simulink model "virtual_world_first_scenario_modified_1"  (R2015b)
settings: Solver=VariableStepAuto  StartTime=start_time  StopTime=stop_time  RelTol=1e-3
values from neighbouring files (symbols this model uses):
  colorFirstCar = [255 0 0]    [virtual_world_script.m]
  colorSecondCar = [0.88 0.95 0.0]    [virtual_world_script.m]
  distanceAmongCars = [0 0 2]    [virtual_world_script.m]
  observer_position = [z_pross y_pross x_pross]    [simulazione_sistema.m]    (also in virtual_world.m = [z_next y_next x_next]; virtual_world_script.m = [z_next y_next x_next])
  rotation_matrix = R_1 * R_2 * R_3    [simulazione_sistema.m]    (also in virtual_world.m = R_z * R_y * R_x; virtual_world_script.m = R_z * R_y * R_x)
  simulationStep = 0.05    [simulation_parameters.m]
libraries: vrlib x50, visionsinks x1
settings Model: ExtModeArmWhenConnect=off  Creator=Giuseppe Silano  LastModifiedBy=giuse
settings DataIOCC: SaveFormat=Array  SignalLoggingName=sigsOut
settings OptimizationCC: BooleanDataType=off  OptimizeBlockIOStorage=off  BufferReuse=off  GlobalBufferReuse=off  ExpressionFolding=off  ExpressionDepthLimit=2147483647  LocalBlockOutputs=off  InitFltsAndDblsToZero=on
settings DebuggingCC: UnderspecifiedInitializationDetection=Classic  MergeDetectMultiDrivingBlocksExec=none  CheckExecutionContextPreStartOutputMsg=on  CheckExecutionContextRuntimeOutputMsg=on  SignalResolutionControl=TryResolveAllWithWarning  MultiTaskDSMMsg=warning  MultiTaskCondExecSysMsg=none  FcnCallInpInsideContextMsg=UseLocalSettings  StateNameClashWarn=warning
settings HardwareCC: ProdBitPerPointer=32  ProdLargestAtomicFloat=None  ProdIntDivRoundTo=Undefined  ProdEndianess=Unspecified  ProdWordSize=32  ProdHWDeviceType=32-bit Generic
settings RTWCC: RetainRTWFile=on
settings GRTTargetCC: TargetFcnLib=ansi_tfl_tmw.mat  GeneratePreprocessorConditionals=Disable all  CombineOutputUpdateFcns=off  GRTInterface=on
settings ConfigComp: CovModelRefEnable=Off  CovSFcnEnable=off

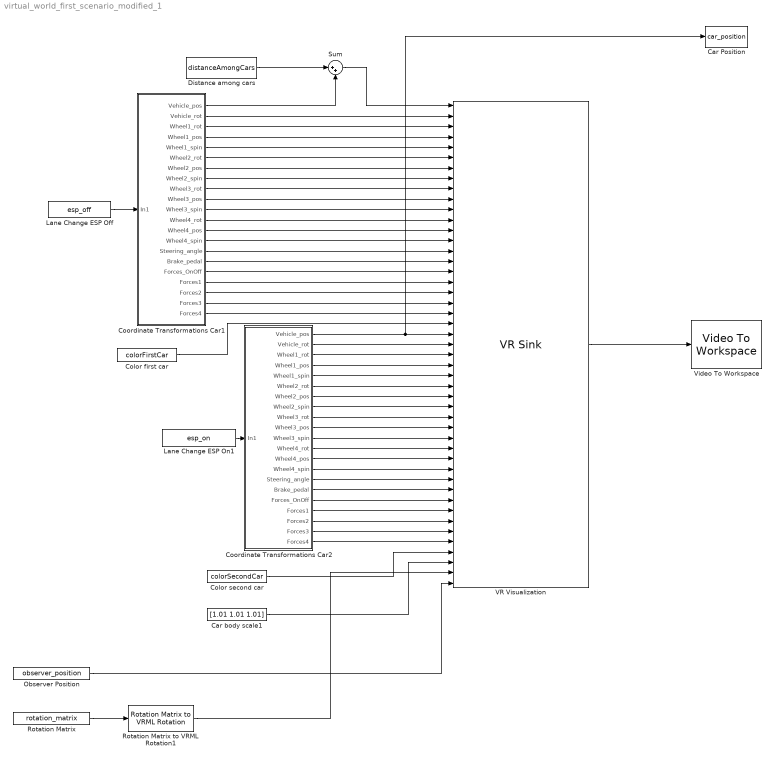
== system virtual_world_first_scenario_modified_1 ==
  Car Position : ToWorkspace  VariableName=car_position  SampleTime=-1
      settings: MaxDataPoints=1
  Car body scale1 : Constant  Value=[1.01 1.01 1.01]
  Color first car : Constant  Value=colorFirstCar
  Color second car : Constant  Value=colorSecondCar
  Coordinate Transformations Car1 : Subsystem
  Coordinate Transformations Car2 : Subsystem
  Distance among cars : Constant  Value=distanceAmongCars
  Lane Change ESP On1 : FromWorkspace  VariableName=esp_on  SampleTime=simulationStep  OutputAfterFinalValue=Holding final value
  "Lane Change ESP Off " : FromWorkspace  VariableName=esp_off  SampleTime=simulationStep  OutputAfterFinalValue=Holding final value
  Observer Position : Constant  Value=observer_position
  Rotation Matrix : Constant  Value=rotation_matrix
  Rotation Matrix to VRML Rotation1 : vrlib/Utilities/Rotation Matrix to VRML Rotation  maxzero=1e-12
  Sum : Sum  Inputs=|++
  VR Visualization : vrlib/VR Sink  InstantiateOnLoad=on  SampleTime=-1  ViewEnable=on  RemoteChange=off  RemoteView=on  FieldsWritten=Car_1.Car_Position.3.1.1.double#Car_1.Car_Rotation.4.1.1.double#Car_1.WheelFL_Rotation.4.1.1.double#Car_1.WheelFL_Translation.3.1.1.double#Car_1.WheelFL_Spin_Rotation.4.1.1.double#Car_1.WheelFR_Rotation.4.1.1.double#Car_1.WheelFR_Translation.3.1.1.double#Car_1.WheelFR_Spin_Rotation.4.1.1.double#Car_1.WheelRL_Rotation.4.1.1.double#Car_1.WheelRL_Translation.3.1.1.double#Car_1.WheelRL_Spin_Rotation.4.1.1.double#Car_1.WheelRR_Rotation.4.1.1.double#Car_1.WheelRR_Translation.3.1.1.double#Car_1.WheelRR_Spin_Rotation.4.1.1.double#Car_1.SteeringWheel1_Rotation.4.1.1.double#Car_1.Backlights_Switch.1.1.1.double#Car_1.Forces_Switch.1.1.1.double#Car_1.Force1_Scale.3.1.1.double#Car_1.Force2_Scale.3.1.1.double#Car_1.Force3_Scale.3.1.1.double#Car_1.Force4_Scale.3.1.1.double#Car_1.Car_DiffuseColor.3.1.1.double#Car_2.Car_Position.3.1.1.double#Car_2.Car_Rotation.4.1.1.double#Car_2.WheelFL_Rotation.4.1.1.double#Car_2.WheelFL_Translation.3.1.1.double#Car_2.WheelFL_Spin_Rotation.4.1.1.double#Car_2.WheelFR_Rotation.4.1.1.double#Car_2.WheelFR_Translation.3.1.1.double#Car_2.WheelFR_Spin_Rotation.4.1.1.double#Car_2.WheelRL_Rotation.4.1.1.double#Car_2.WheelRL_Translation.3.1.1.double#Car_2.WheelRL_Spin_Rotation.4.1.1.double#Car_2.WheelRR_Rotation.4.1.1.double#Car_2.WheelRR_Translation.3.1.1.double#Car_2.WheelRR_Spin_Rotation.4.1.1.double#Car_2.SteeringWheel1_Rotation.4.1.1.double#Car_2.Backlights_Switch.1.1.1.double#Car_2.Forces_Switch.1.1.1.double#Car_2.Force1_Scale.3.1.1.double#Car_2.Force2_Scale.3.1.1.double#Car_2.Force3_Scale.3.1.1.double#Car_2.Force4_Scale.3.1.1.double#Car_2.Car_DiffuseColor.3.1.1.double#Car_2.Body_Scale.3.1.1.double#FlyingCamera.orientation.4.1.1.double#FlyingCamera.position.3.1.1.double  WorldFileName=octavia_scene_lchg_2cars_modified_scenario_1.wrl  WorldDescription=Vehicle Dynamics Visualization - Multiple Vehicles  AutoView=on  VideoDimensions=[800 600]  AllowVariableSize=off  FigureProperties="{'Position', 'Name', 'Viewpoint', 'CameraBound', 'CameraDirection', 'CameraPosition', 'CameraUpVector', 'ZoomFactor', 'Antialiasing', 'Headlight', 'Lighting', 'NavPanel', 'Sound', 'StatusBar', 'Stereo3D', 'Stereo3DCameraOffset', 'Stereo3DHIT', 'ToolBar', 'Textures', 'Transparency', 'Triad', 'Wireframe', 'NavZones', 'NavMode', 'NavSpeed', 'CaptureFileFormat', 'CaptureFileName', 'Record2DCompressMethod', 'Record2DCompressQuality', 'Record2D', 'Record2DFileName', 'Record2DFPS'; [1.5200000000000000e+02   2.4800000000000000e+02   5.7600000000000000e+02   3.8000000000000000e+02], 'Vehicle Dynamics Visualization - Multiple Vehicles', 'Car - View from Right Above Ahead', 'on', [0.0000000000000000e+00   0.0000000000000000e+00  -1.0000000000000000e+00], [0.0000000000000000e+00   0.0000000000000000e+00   0.0000000000000000e+00], [0.0000000000000000e+00   1.0000000000000000e+00   0.0000000000000000e+00], [1.0000000000000000e+00], 'on', 'off', 'on', 'halfbar', 'on', 'on', 'off', [1.0000000149011612e-01], [0.0000000000000000e+00], 'on', 'on', 'on', 'none', 'off', 'off', 'walk', 'normal', 'tif', '%f_anim_%n.tif', 'auto', [7.5000000000000000e+01], 'off', '%f_anim_%n.avi', 'auto'; [7.3300000000000000e+02   6.0000000000000000e+01   6.0000000000000000e+02   8.0000000000000000e+02], 'Vehicle Dynamics Visualization - Multiple Vehicles', 'External observer: drone', 'on', [0.0000000000000000e+00   0.0000000000000000e+00  -1.0000000000000000e+00], [0.0000000000000000e+00   0.0000000000000000e+00   0.0000000000000000e+00], [0.0000000000000000e+00   1.0000000000000000e+00   0.0000000000000000e+00], [1.0000000000000000e+00], 'on', 'off', 'on', 'none', 'on', 'off', 'off', [1.0000000149011612e-01], [0.0000000000000000e+00], 'off', 'on', 'on', 'none', 'off', 'off', 'walk', 'normal', 'tif', '%f_anim_%n.tif', 'auto', [7.5000000000000000e+01], 'off', '***video***', 'auto'}"
  Video To Workspace : visionsinks/Video To Workspace  VariableName=image  NumInputs=1  DataLimit=1  DecimationFactor=1  LogFi=off  InPortLabels=R|G|B
  wires:
  VR Visualization/1 -> Video To Workspace/1
  "Lane Change ESP Off "/1 -> Coordinate Transformations Car1/1(In1)
  Lane Change ESP On1/1 -> Coordinate Transformations Car2/1(In1)
  Rotation Matrix/1 -> Rotation Matrix to VRML Rotation1/1
  Distance among cars/1 -> Sum/1
  Coordinate Transformations Car1/2(Vehicle_rot) -> VR Visualization/2
  Coordinate Transformations Car1/3(Wheel1_rot) -> VR Visualization/3
  Coordinate Transformations Car1/4(Wheel1_pos) -> VR Visualization/4
  Coordinate Transformations Car1/5(Wheel1_spin) -> VR Visualization/5
  Coordinate Transformations Car1/6(Wheel2_rot) -> VR Visualization/6
  Coordinate Transformations Car1/7(Wheel2_pos) -> VR Visualization/7
  Coordinate Transformations Car1/8(Wheel2_spin) -> VR Visualization/8
  Coordinate Transformations Car1/9(Wheel3_rot) -> VR Visualization/9
  Coordinate Transformations Car1/10(Wheel3_pos) -> VR Visualization/10
  Coordinate Transformations Car1/11(Wheel3_spin) -> VR Visualization/11
  Coordinate Transformations Car1/12(Wheel4_rot) -> VR Visualization/12
  Coordinate Transformations Car1/13(Wheel4_pos) -> VR Visualization/13
  Coordinate Transformations Car1/14(Wheel4_spin) -> VR Visualization/14
  Coordinate Transformations Car1/15(Steering_angle) -> VR Visualization/15
  Coordinate Transformations Car1/16(Brake_pedal) -> VR Visualization/16
  Coordinate Transformations Car1/17(Forces_OnOff) -> VR Visualization/17
  Coordinate Transformations Car1/18(Forces1) -> VR Visualization/18
  Coordinate Transformations Car1/19(Forces2) -> VR Visualization/19
  Coordinate Transformations Car1/20(Forces3) -> VR Visualization/20
  Coordinate Transformations Car1/21(Forces4) -> VR Visualization/21
  Color first car/1 -> VR Visualization/22
  Coordinate Transformations Car2/2(Vehicle_rot) -> VR Visualization/24
  Coordinate Transformations Car2/3(Wheel1_rot) -> VR Visualization/25
  Coordinate Transformations Car2/4(Wheel1_pos) -> VR Visualization/26
  Coordinate Transformations Car2/5(Wheel1_spin) -> VR Visualization/27
  Coordinate Transformations Car2/6(Wheel2_rot) -> VR Visualization/28
  Coordinate Transformations Car2/7(Wheel2_pos) -> VR Visualization/29
  Coordinate Transformations Car2/8(Wheel2_spin) -> VR Visualization/30
  Coordinate Transformations Car2/9(Wheel3_rot) -> VR Visualization/31
  Coordinate Transformations Car2/10(Wheel3_pos) -> VR Visualization/32
  Coordinate Transformations Car2/11(Wheel3_spin) -> VR Visualization/33
  Coordinate Transformations Car2/12(Wheel4_rot) -> VR Visualization/34
  Coordinate Transformations Car2/13(Wheel4_pos) -> VR Visualization/35
  Coordinate Transformations Car2/14(Wheel4_spin) -> VR Visualization/36
  Coordinate Transformations Car2/15(Steering_angle) -> VR Visualization/37
  Coordinate Transformations Car2/16(Brake_pedal) -> VR Visualization/38
  Coordinate Transformations Car2/17(Forces_OnOff) -> VR Visualization/39
  Coordinate Transformations Car2/18(Forces1) -> VR Visualization/40
  Coordinate Transformations Car2/19(Forces2) -> VR Visualization/41
  Coordinate Transformations Car2/20(Forces3) -> VR Visualization/42
  Coordinate Transformations Car2/21(Forces4) -> VR Visualization/43
  Color second car/1 -> VR Visualization/44
  Car body scale1/1 -> VR Visualization/45
  Rotation Matrix to VRML Rotation1/1 -> VR Visualization/46
  Observer Position/1 -> VR Visualization/47
  Coordinate Transformations Car2/1(Vehicle_pos) -> Car Position/1, VR Visualization/23
  Coordinate Transformations Car1/1(Vehicle_pos) -> Sum/2
  Sum/1 -> VR Visualization/1

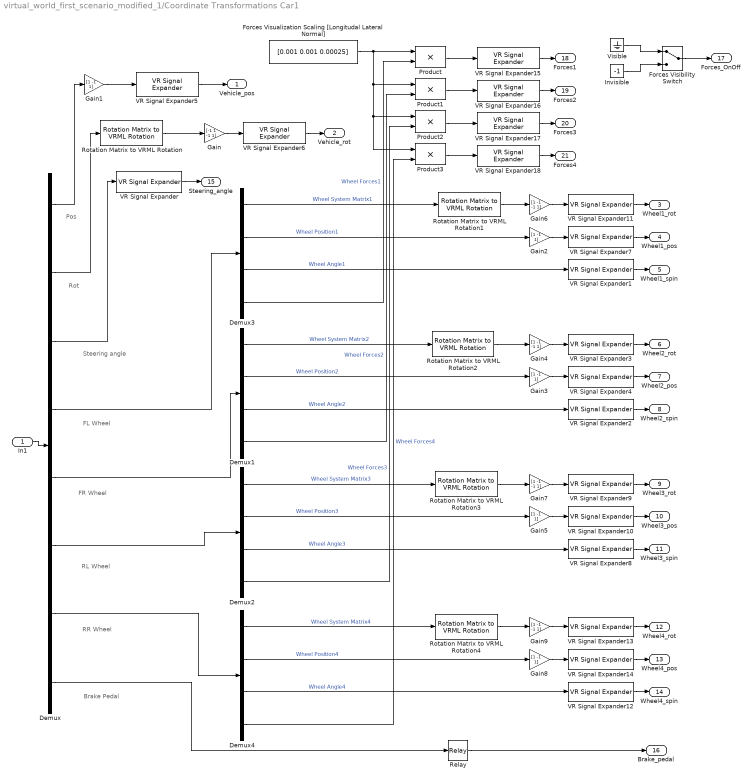
== system virtual_world_first_scenario_modified_1/Coordinate Transformations Car1 ==
  note: Steering angle
  note: FL Wheel
  note: FR Wheel
  note: RL Wheel
  note: RR Wheel
  note: Brake Pedal
  note: Pos
  note: Rot
  In1 : Inport
  Demux : Demux  Outputs=[3,9,1,16,16,16,16,1]
  Demux{1..4} (4 alike) : Demux  Outputs=[9,3,1,3]
  Forces Visibility Switch : ManualSwitch
  Forces Visualization Scaling [Longitudal Lateral Normal] : Constant  Value=[0.001 0.001 0.00025]
  Gain : Gain  Gain=[-1 1 -1 1]  SaturateOnIntegerOverflow=on  OutDataTypeStr=Inherit: Same as input  ParamDataTypeStr=Inherit: Same as input
  Gain{1..3,5,8} (5 alike) : Gain  Gain=[1 -1 1]  SaturateOnIntegerOverflow=on  OutDataTypeStr=Inherit: Same as input  ParamDataTypeStr=Inherit: Same as input
  Gain{4,6..7,9} (4 alike) : Gain  Gain=[1 -1 -1 1]  SaturateOnIntegerOverflow=on  OutDataTypeStr=Inherit: Same as input  ParamDataTypeStr=Inherit: Same as input
  Invisible : Constant  Value=-1
  Product{,1..3} (4 alike) : Product  SaturateOnIntegerOverflow=on  OutDataTypeStr=Inherit: Same as first input
  Relay : Relay
  Rotation Matrix to VRML Rotation{,1..4} (5 alike) : vrlib/Utilities/Rotation Matrix to VRML Rotation  maxzero=1e-12
  VR Signal Expander{,1..2,8,12} (5 alike) : vrlib/VR Signal Expander  outwidth=4  outidx=[4]
  VR Signal Expander{4,7,10,14} (4 alike) : vrlib/VR Signal Expander  outwidth=3  outidx=[1 3 2 ]
  VR Signal Expander{3,6,9,11,13} (5 alike) : vrlib/VR Signal Expander  outwidth=4  outidx=[1 3 2 4]
  VR Signal Expander{5,15..18} (5 alike) : vrlib/VR Signal Expander  outwidth=3  outidx=[1 3 2]
  Visible : Ground
  Vehicle_pos : Outport
  Vehicle_rot : Outport  Port=2
  Wheel1_rot : Outport  Port=3
  Wheel1_pos : Outport  Port=4
  Wheel1_spin : Outport  Port=5
  Wheel2_rot : Outport  Port=6
  Wheel2_pos : Outport  Port=7
  Wheel2_spin : Outport  Port=8
  Wheel3_rot : Outport  Port=9
  Wheel3_pos : Outport  Port=10
  Wheel3_spin : Outport  Port=11
  Wheel4_rot : Outport  Port=12
  Wheel4_pos : Outport  Port=13
  Wheel4_spin : Outport  Port=14
  Steering_angle : Outport  Port=15
  Brake_pedal : Outport  Port=16
  Forces_OnOff : Outport  Port=17
  Forces1 : Outport  Port=18
  Forces2 : Outport  Port=19
  Forces3 : Outport  Port=20
  Forces4 : Outport  Port=21
  wires:
  Gain1/1 -> VR Signal Expander5/1
  Rotation Matrix to VRML Rotation/1 -> Gain/1
  Gain/1 -> VR Signal Expander6/1
  Gain6/1 -> VR Signal Expander11/1
  Gain2/1 -> VR Signal Expander7/1
  Demux3/1 -> Rotation Matrix to VRML Rotation1/1  "Wheel System Matrix1"
  Demux3/2 -> Gain2/1  "Wheel Position1"
  Demux3/3 -> VR Signal Expander1/1  "Wheel Angle1"
  Gain4/1 -> VR Signal Expander3/1
  Rotation Matrix to VRML Rotation2/1 -> Gain4/1
  Gain3/1 -> VR Signal Expander4/1
  Demux1/1 -> Rotation Matrix to VRML Rotation2/1  "Wheel System Matrix2"
  Demux1/2 -> Gain3/1  "Wheel Position2"
  Demux1/3 -> VR Signal Expander2/1  "Wheel Angle2"
  Gain7/1 -> VR Signal Expander9/1
  Rotation Matrix to VRML Rotation3/1 -> Gain7/1
  Demux2/4 -> Product2/2  "Wheel Forces3"
  Gain5/1 -> VR Signal Expander10/1
  Demux2/1 -> Rotation Matrix to VRML Rotation3/1  "Wheel System Matrix3"
  Demux2/2 -> Gain5/1  "Wheel Position3"
  Demux2/3 -> VR Signal Expander8/1  "Wheel Angle3"
  Gain9/1 -> VR Signal Expander13/1
  Rotation Matrix to VRML Rotation4/1 -> Gain9/1
  Demux4/4 -> Product3/2  "Wheel Forces4"
  Gain8/1 -> VR Signal Expander14/1
  Demux4/1 -> Rotation Matrix to VRML Rotation4/1  "Wheel System Matrix4"
  Demux4/2 -> Gain8/1  "Wheel Position4"
  Demux4/3 -> VR Signal Expander12/1  "Wheel Angle4"
  VR Signal Expander5/1 -> Vehicle_pos/1
  Demux3/4 -> Product/2  "Wheel Forces1"
  Demux1/4 -> Product1/2  "Wheel Forces2"
  Product/1 -> VR Signal Expander15/1
  Product1/1 -> VR Signal Expander16/1
  Product2/1 -> VR Signal Expander17/1
  Product3/1 -> VR Signal Expander18/1
  VR Signal Expander6/1 -> Vehicle_rot/1
  VR Signal Expander15/1 -> Forces1/1
  VR Signal Expander16/1 -> Forces2/1
  VR Signal Expander17/1 -> Forces3/1
  VR Signal Expander18/1 -> Forces4/1
  VR Signal Expander/1 -> Steering_angle/1
  VR Signal Expander11/1 -> Wheel1_rot/1
  In1/1 -> Demux/1
  VR Signal Expander7/1 -> Wheel1_pos/1
  VR Signal Expander1/1 -> Wheel1_spin/1
  VR Signal Expander3/1 -> Wheel2_rot/1
  VR Signal Expander4/1 -> Wheel2_pos/1
  VR Signal Expander2/1 -> Wheel2_spin/1
  VR Signal Expander9/1 -> Wheel3_rot/1
  VR Signal Expander10/1 -> Wheel3_pos/1
  VR Signal Expander8/1 -> Wheel3_spin/1
  VR Signal Expander13/1 -> Wheel4_rot/1
  VR Signal Expander14/1 -> Wheel4_pos/1
  VR Signal Expander12/1 -> Wheel4_spin/1
  Demux/8 -> Relay/1
  Relay/1 -> Brake_pedal/1
  Demux/1 -> Gain1/1
  Demux/2 -> Rotation Matrix to VRML Rotation/1
  Demux/3 -> VR Signal Expander/1
  Demux/4 -> Demux3/1
  Demux/5 -> Demux1/1
  Demux/6 -> Demux2/1
  Demux/7 -> Demux4/1
  Forces Visualization Scaling [Longitudal Lateral Normal]/1 -> Product/1, Product1/1, Product2/1, Product3/1
  Rotation Matrix to VRML Rotation1/1 -> Gain6/1
  Visible/1 -> Forces Visibility Switch/1
  Invisible/1 -> Forces Visibility Switch/2
  Forces Visibility Switch/1 -> Forces_OnOff/1

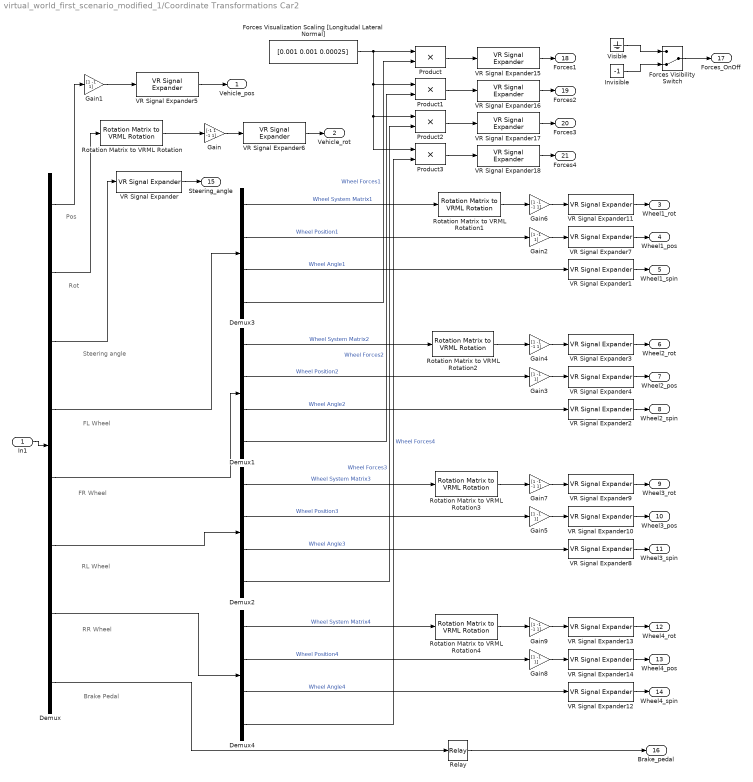
== system virtual_world_first_scenario_modified_1/Coordinate Transformations Car2 ==
  note: Steering angle
  note: FL Wheel
  note: FR Wheel
  note: RL Wheel
  note: RR Wheel
  note: Brake Pedal
  note: Pos
  note: Rot
  In1 : Inport
  Demux : Demux  Outputs=[3,9,1,16,16,16,16,1]
  Demux{1..4} (4 alike) : Demux  Outputs=[9,3,1,3]
  Forces Visibility Switch : ManualSwitch  CurrentSetting=0
  Forces Visualization Scaling [Longitudal Lateral Normal] : Constant  Value=[0.001 0.001 0.00025]
  Gain : Gain  Gain=[-1 1 -1 1]  SaturateOnIntegerOverflow=on  OutDataTypeStr=Inherit: Same as input  ParamDataTypeStr=Inherit: Same as input
  Gain{1..3,5,8} (5 alike) : Gain  Gain=[1 -1 1]  SaturateOnIntegerOverflow=on  OutDataTypeStr=Inherit: Same as input  ParamDataTypeStr=Inherit: Same as input
  Gain{4,6..7,9} (4 alike) : Gain  Gain=[1 -1 -1 1]  SaturateOnIntegerOverflow=on  OutDataTypeStr=Inherit: Same as input  ParamDataTypeStr=Inherit: Same as input
  Invisible : Constant  Value=-1
  Product{,1..3} (4 alike) : Product  SaturateOnIntegerOverflow=on  OutDataTypeStr=Inherit: Same as first input
  Relay : Relay
  Rotation Matrix to VRML Rotation{,1..4} (5 alike) : vrlib/Utilities/Rotation Matrix to VRML Rotation  maxzero=1e-12
  VR Signal Expander{,1..2,8,12} (5 alike) : vrlib/VR Signal Expander  outwidth=4  outidx=[4]
  VR Signal Expander{4,7,10,14} (4 alike) : vrlib/VR Signal Expander  outwidth=3  outidx=[1 3 2 ]
  VR Signal Expander{3,6,9,11,13} (5 alike) : vrlib/VR Signal Expander  outwidth=4  outidx=[1 3 2 4]
  VR Signal Expander{5,15..18} (5 alike) : vrlib/VR Signal Expander  outwidth=3  outidx=[1 3 2]
  Visible : Ground
  Vehicle_pos : Outport
  Vehicle_rot : Outport  Port=2
  Wheel1_rot : Outport  Port=3
  Wheel1_pos : Outport  Port=4
  Wheel1_spin : Outport  Port=5
  Wheel2_rot : Outport  Port=6
  Wheel2_pos : Outport  Port=7
  Wheel2_spin : Outport  Port=8
  Wheel3_rot : Outport  Port=9
  Wheel3_pos : Outport  Port=10
  Wheel3_spin : Outport  Port=11
  Wheel4_rot : Outport  Port=12
  Wheel4_pos : Outport  Port=13
  Wheel4_spin : Outport  Port=14
  Steering_angle : Outport  Port=15
  Brake_pedal : Outport  Port=16
  Forces_OnOff : Outport  Port=17
  Forces1 : Outport  Port=18
  Forces2 : Outport  Port=19
  Forces3 : Outport  Port=20
  Forces4 : Outport  Port=21
  wires:
  Gain1/1 -> VR Signal Expander5/1
  Rotation Matrix to VRML Rotation/1 -> Gain/1
  Gain/1 -> VR Signal Expander6/1
  Gain6/1 -> VR Signal Expander11/1
  Gain2/1 -> VR Signal Expander7/1
  Demux3/1 -> Rotation Matrix to VRML Rotation1/1  "Wheel System Matrix1"
  Demux3/2 -> Gain2/1  "Wheel Position1"
  Demux3/3 -> VR Signal Expander1/1  "Wheel Angle1"
  Gain4/1 -> VR Signal Expander3/1
  Rotation Matrix to VRML Rotation2/1 -> Gain4/1
  Gain3/1 -> VR Signal Expander4/1
  Demux1/1 -> Rotation Matrix to VRML Rotation2/1  "Wheel System Matrix2"
  Demux1/2 -> Gain3/1  "Wheel Position2"
  Demux1/3 -> VR Signal Expander2/1  "Wheel Angle2"
  Gain7/1 -> VR Signal Expander9/1
  Rotation Matrix to VRML Rotation3/1 -> Gain7/1
  Demux2/4 -> Product2/2  "Wheel Forces3"
  Gain5/1 -> VR Signal Expander10/1
  Demux2/1 -> Rotation Matrix to VRML Rotation3/1  "Wheel System Matrix3"
  Demux2/2 -> Gain5/1  "Wheel Position3"
  Demux2/3 -> VR Signal Expander8/1  "Wheel Angle3"
  Gain9/1 -> VR Signal Expander13/1
  Rotation Matrix to VRML Rotation4/1 -> Gain9/1
  Demux4/4 -> Product3/2  "Wheel Forces4"
  Gain8/1 -> VR Signal Expander14/1
  Demux4/1 -> Rotation Matrix to VRML Rotation4/1  "Wheel System Matrix4"
  Demux4/2 -> Gain8/1  "Wheel Position4"
  Demux4/3 -> VR Signal Expander12/1  "Wheel Angle4"
  VR Signal Expander5/1 -> Vehicle_pos/1
  Demux3/4 -> Product/2  "Wheel Forces1"
  Demux1/4 -> Product1/2  "Wheel Forces2"
  Product/1 -> VR Signal Expander15/1
  Product1/1 -> VR Signal Expander16/1
  Product2/1 -> VR Signal Expander17/1
  Product3/1 -> VR Signal Expander18/1
  VR Signal Expander6/1 -> Vehicle_rot/1
  VR Signal Expander15/1 -> Forces1/1
  VR Signal Expander16/1 -> Forces2/1
  VR Signal Expander17/1 -> Forces3/1
  VR Signal Expander18/1 -> Forces4/1
  VR Signal Expander/1 -> Steering_angle/1
  VR Signal Expander11/1 -> Wheel1_rot/1
  In1/1 -> Demux/1
  VR Signal Expander7/1 -> Wheel1_pos/1
  VR Signal Expander1/1 -> Wheel1_spin/1
  VR Signal Expander3/1 -> Wheel2_rot/1
  VR Signal Expander4/1 -> Wheel2_pos/1
  VR Signal Expander2/1 -> Wheel2_spin/1
  VR Signal Expander9/1 -> Wheel3_rot/1
  VR Signal Expander10/1 -> Wheel3_pos/1
  VR Signal Expander8/1 -> Wheel3_spin/1
  VR Signal Expander13/1 -> Wheel4_rot/1
  VR Signal Expander14/1 -> Wheel4_pos/1
  VR Signal Expander12/1 -> Wheel4_spin/1
  Demux/8 -> Relay/1
  Relay/1 -> Brake_pedal/1
  Demux/1 -> Gain1/1
  Demux/2 -> Rotation Matrix to VRML Rotation/1
  Demux/3 -> VR Signal Expander/1
  Demux/4 -> Demux3/1
  Demux/5 -> Demux1/1
  Demux/6 -> Demux2/1
  Demux/7 -> Demux4/1
  Forces Visualization Scaling [Longitudal Lateral Normal]/1 -> Product/1, Product1/1, Product2/1, Product3/1
  Rotation Matrix to VRML Rotation1/1 -> Gain6/1
  Visible/1 -> Forces Visibility Switch/1
  Invisible/1 -> Forces Visibility Switch/2
  Forces Visibility Switch/1 -> Forces_OnOff/1
